simulink model "double_pendulum_model"  (R2018a)
settings: Solver=VariableStepAuto  StartTime=0.0  StopTime=30  RelTol=1e-3
undefined symbols (not defined in the file): params
settings Model: Creator=dramih  LastModifiedBy=dramih

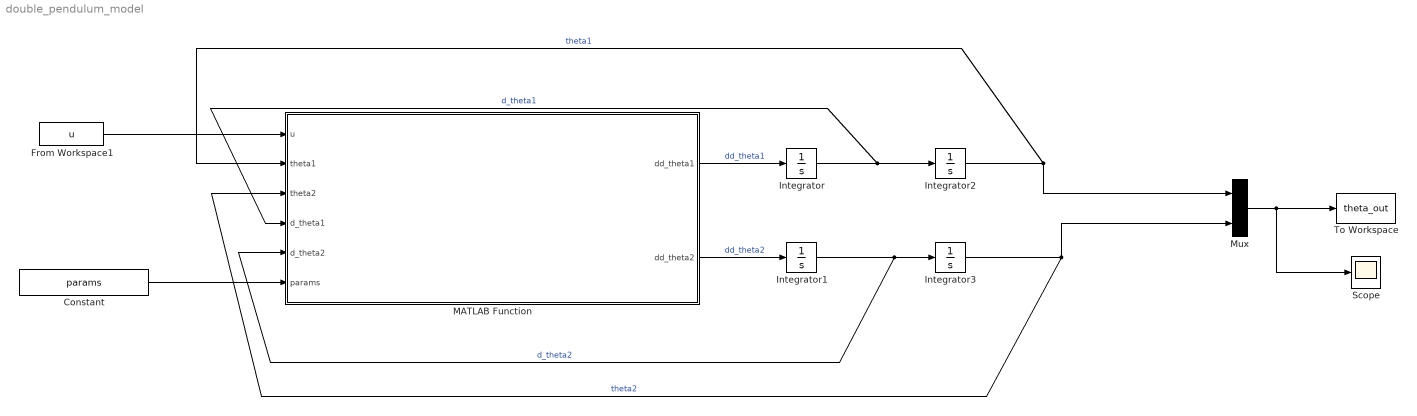
== system double_pendulum_model ==
  Constant : Constant  Value=params  OutDataTypeStr=Bus: params_bus
  From Workspace1 : FromWorkspace  VariableName=u  SampleTime=0
  Integrator{,1..3} (4 alike) : Integrator
  MATLAB Function : MATLAB Function  TreatAsAtomicUnit=on
  Mux : Mux  Inputs=2
  Scope : Scope
  To Workspace : ToWorkspace  VariableName=theta_out  SaveFormat=Timeseries  SampleTime=-1
  wires:
  MATLAB Function/1(dd_theta1) -> Integrator/1  "dd_theta1"
  MATLAB Function/2(dd_theta2) -> Integrator1/1  "dd_theta2"
  Integrator/1 -> MATLAB Function/4(d_theta1), Integrator2/1  "d_theta1"
  Integrator1/1 -> MATLAB Function/5(d_theta2), Integrator3/1  "d_theta2"
  Integrator2/1 -> Mux/1, MATLAB Function/2(theta1)  "theta1"
  Integrator3/1 -> Mux/2, MATLAB Function/3(theta2)  "theta2"
  From Workspace1/1 -> MATLAB Function/1(u)
  Constant/1 -> MATLAB Function/6(params)
  Mux/1 -> Scope/1, To Workspace/1

== matlab function double_pendulum_model/MATLAB Function ==
  data: u input; theta1 input; theta2 input; d_theta1 input; d_theta2 input; dd_theta1 output; dd_theta2 output; params input
function [dd_theta1, dd_theta2] = fcn(u, theta1, theta2, d_theta1, d_theta2, params)


A = -(d_theta2^2) * sin(theta1 - theta2) - 2 * (params.g / params.l) * sin(theta1) - params.zeta * d_theta1 + (1 / (params.m * params.l^2)) * u;

B = (d_theta1^2) * sin(theta1 - theta2) - (params.g / params.l) * sin(theta2) - params.zeta * d_theta2;



dd_theta1 = (B * cos(theta1 - theta2) - A) / (-cos(2 * (theta1 - theta2)));

dd_theta2 = (2 * B - A * cos(theta1 - theta2)) / (cos(2 * (theta1 - theta2)));



end
